simulink model "coif1_5_Level"  (R2021a)
settings: Solver=VariableStepAuto  StartTime=0.0  StopTime=8  RelTol=1e-3
undefined symbols (not defined in the file): lambda2
libraries: dspsigops x11, dspquant2 x1
(part 2 of 3)

== system coif1_5_Level/2nd_Level_Decomp/LoD_Even ==
  In_LoD_e : Inport  OutDataTypeStr=double  SampleTime=1/44100
  Add : Sum  AccumDataTypeStr=double  OutDataTypeStr=double  LockScale=on
  Add1 : Sum  AccumDataTypeStr=double  OutDataTypeStr=double  LockScale=on
  Delay{,1..3} (4 alike) : Delay  DelayLength=1  SampleTime=1/44100
  LoD_0 : Constant  Value=-0.015655728  OutDataTypeStr=double  SampleTime=1/44100
  LoD_2 : Constant  Value=0.384864847  OutDataTypeStr=double  SampleTime=1/44100
  LoD_4 : Constant  Value=0.337897662  OutDataTypeStr=double  SampleTime=1/44100
  Multiply : Product  OutDataTypeStr=double  LockScale=on
  Multiply1 : Product  OutDataTypeStr=double  LockScale=on
  Multiply2 : Product  OutDataTypeStr=double  LockScale=on
  Rate Transition : RateTransition  OutPortSampleTime=1/44100
  Rate Transition1 : RateTransition  OutPortSampleTime=1/44100
  Out_LoD_e : Outport  OutDataTypeStr=double  SampleTime=1/44100  VectorParamsAs1DForOutWhenUnconnected=off
  wires:
  In_LoD_e/1 -> Delay/1, Multiply/2
  Delay3/1 -> Add/2
  LoD_2/1 -> Multiply1/1
  Multiply/1 -> Add/1
  Rate Transition/1 -> Delay1/1, Multiply1/2
  LoD_4/1 -> Multiply2/1
  Delay2/1 -> Add1/2
  Multiply1/1 -> Add1/1
  Multiply2/1 -> Delay2/1
  Add1/1 -> Delay3/1
  Rate Transition1/1 -> Multiply2/2
  Add/1 -> Out_LoD_e/1
  Delay1/1 -> Rate Transition1/1
  LoD_0/1 -> Multiply/1
  Delay/1 -> Rate Transition/1

== system coif1_5_Level/2nd_Level_Decomp/LoD_Odd ==
  In_LoD_o : Inport  OutDataTypeStr=double  SampleTime=1/44100
  Add : Sum  AccumDataTypeStr=double  OutDataTypeStr=double  LockScale=on
  Add1 : Sum  AccumDataTypeStr=double  OutDataTypeStr=double  LockScale=on
  Delay{,1..3} (4 alike) : Delay  DelayLength=1  SampleTime=1/44100
  LoD_1 : Constant  Value=-0.07273262  OutDataTypeStr=double  SampleTime=1/44100
  LoD_3 : Constant  Value=0.85257202  OutDataTypeStr=double  SampleTime=1/44100
  LoD_5 : Constant  Value=-0.07273262  OutDataTypeStr=double  SampleTime=1/44100
  Multiply : Product  OutDataTypeStr=double  LockScale=on
  Multiply1 : Product  OutDataTypeStr=double  LockScale=on
  Multiply2 : Product  OutDataTypeStr=double  LockScale=on
  Rate Transition : RateTransition  OutPortSampleTime=1/44100
  Rate Transition1 : RateTransition  OutPortSampleTime=1/44100
  Out_LoD_o : Outport  OutDataTypeStr=double  SampleTime=1/44100  VectorParamsAs1DForOutWhenUnconnected=off
  wires:
  In_LoD_o/1 -> Delay/1, Multiply/2
  Delay3/1 -> Add/2
  LoD_3/1 -> Multiply1/1
  Delay/1 -> Rate Transition/1
  Multiply/1 -> Add/1
  Rate Transition/1 -> Delay1/1, Multiply1/2
  LoD_5/1 -> Multiply2/1
  Delay2/1 -> Add1/2
  Multiply1/1 -> Add1/1
  Multiply2/1 -> Delay2/1
  Add1/1 -> Delay3/1
  Rate Transition1/1 -> Multiply2/2
  Add/1 -> Out_LoD_o/1
  Delay1/1 -> Rate Transition1/1
  LoD_1/1 -> Multiply/1

== system coif1_5_Level/2nd_Level_Recon/HiR_Even1 ==
  In_HiR_e : Inport  OutDataTypeStr=double  SampleTime=1/44100
  Add : Sum  AccumDataTypeStr=double  OutDataTypeStr=double  LockScale=on
  Add1 : Sum  AccumDataTypeStr=double  OutDataTypeStr=double  LockScale=on
  Delay{,1..3} (4 alike) : Delay  DelayLength=1  SampleTime=1/44100
  HiR_0 : Constant  Value=-0.015655728  OutDataTypeStr=double  SampleTime=1/44100
  HiR_2 : Constant  Value=0.384864847  OutDataTypeStr=double  SampleTime=1/44100
  HiR_4 : Constant  Value=0.337897662  OutDataTypeStr=double  SampleTime=1/44100
  Multiply : Product  OutDataTypeStr=double  LockScale=on
  Multiply1 : Product  OutDataTypeStr=double  LockScale=on
  Multiply2 : Product  OutDataTypeStr=double  LockScale=on
  Rate Transition : RateTransition  OutPortSampleTime=1/44100
  Rate Transition1 : RateTransition  OutPortSampleTime=1/44100
  Out_HiR_e : Outport  OutDataTypeStr=double  SampleTime=1/44100  VectorParamsAs1DForOutWhenUnconnected=off
  wires:
  In_HiR_e/1 -> Multiply/2, Delay/1
  Delay/1 -> Rate Transition/1
  Delay3/1 -> Add/2
  Multiply/1 -> Add/1
  HiR_0/1 -> Multiply/1
  HiR_2/1 -> Multiply1/1
  Rate Transition/1 -> Delay1/1, Multiply1/2
  Add/1 -> Out_HiR_e/1
  Delay1/1 -> Rate Transition1/1
  Rate Transition1/1 -> Multiply2/2
  Multiply2/1 -> Delay2/1
  Delay2/1 -> Add1/2
  Multiply1/1 -> Add1/1
  Add1/1 -> Delay3/1
  HiR_4/1 -> Multiply2/1

== system coif1_5_Level/2nd_Level_Recon/HiR_Odd1 ==
  In_HiR_o : Inport  OutDataTypeStr=double  SampleTime=1/44100
  Add1 : Sum  AccumDataTypeStr=double  OutDataTypeStr=double  LockScale=on
  Add2 : Sum  AccumDataTypeStr=double  OutDataTypeStr=double  LockScale=on
  Delay{1..2,4..5} (4 alike) : Delay  DelayLength=1  SampleTime=1/44100
  HiR_1 : Constant  Value=0.07273262  OutDataTypeStr=double  SampleTime=1/44100
  HiR_3 : Constant  Value=-0.85257202  OutDataTypeStr=double  SampleTime=1/44100
  HiR_5 : Constant  Value=0.07273262  OutDataTypeStr=double  SampleTime=1/44100
  Multiply2 : Product  OutDataTypeStr=double  LockScale=on
  Multiply3 : Product  OutDataTypeStr=double  LockScale=on
  Multiply4 : Product  OutDataTypeStr=double  LockScale=on
  Rate Transition1 : RateTransition  OutPortSampleTime=1/44100
  Rate Transition2 : RateTransition  OutPortSampleTime=1/44100
  Out_HiR_o : Outport  OutDataTypeStr=double  SampleTime=1/44100  VectorParamsAs1DForOutWhenUnconnected=off
  wires:
  HiR_5/1 -> Multiply4/1
  Add1/1 -> Out_HiR_o/1
  Rate Transition2/1 -> Multiply4/2
  Rate Transition1/1 -> Delay2/1, Multiply3/2
  Multiply4/1 -> Delay4/1
  Add2/1 -> Delay5/1
  Multiply3/1 -> Add2/1
  Delay4/1 -> Add2/2
  Multiply2/1 -> Add1/1
  Delay2/1 -> Rate Transition2/1
  In_HiR_o/1 -> Multiply2/2, Delay1/1
  Delay1/1 -> Rate Transition1/1
  Delay5/1 -> Add1/2
  HiR_1/1 -> Multiply2/1
  HiR_3/1 -> Multiply3/1

== system coif1_5_Level/2nd_Level_Recon/LoR_Even1 ==
  In_LoR_e : Inport  OutDataTypeStr=double  SampleTime=1/44100
  Add1 : Sum  AccumDataTypeStr=double  OutDataTypeStr=double  LockScale=on
  Add2 : Sum  AccumDataTypeStr=double  OutDataTypeStr=double  LockScale=on
  Delay{1..2,4..5} (4 alike) : Delay  DelayLength=1  SampleTime=1/44100
  LoR_0 : Constant  Value=-0.07273262  OutDataTypeStr=double  SampleTime=1/44100
  LoR_2 : Constant  Value=0.85257202  OutDataTypeStr=double  SampleTime=1/44100
  LoR_4 : Constant  Value=-0.07273262  OutDataTypeStr=double  SampleTime=1/44100
  Multiply2 : Product  OutDataTypeStr=double  LockScale=on
  Multiply3 : Product  OutDataTypeStr=double  LockScale=on
  Multiply4 : Product  OutDataTypeStr=double  LockScale=on
  Rate Transition1 : RateTransition  OutPortSampleTime=1/44100
  Rate Transition2 : RateTransition  OutPortSampleTime=1/44100
  Out_LoR_e : Outport  OutDataTypeStr=double  SampleTime=1/44100  VectorParamsAs1DForOutWhenUnconnected=off
  wires:
  Add2/1 -> Delay5/1
  Delay2/1 -> Rate Transition2/1
  Add1/1 -> Out_LoR_e/1
  Multiply3/1 -> Add2/1
  Delay5/1 -> Add1/2
  Delay1/1 -> Rate Transition1/1
  Multiply2/1 -> Add1/1
  Delay4/1 -> Add2/2
  Multiply4/1 -> Delay4/1
  Rate Transition2/1 -> Multiply4/2
  In_LoR_e/1 -> Multiply2/2, Delay1/1
  Rate Transition1/1 -> Delay2/1, Multiply3/2
  LoR_4/1 -> Multiply4/1
  LoR_2/1 -> Multiply3/1
  LoR_0/1 -> Multiply2/1

== system coif1_5_Level/2nd_Level_Recon/LoR_Odd1 ==
  In_LoR_o : Inport  OutDataTypeStr=double  SampleTime=1/44100
  Add1 : Sum  AccumDataTypeStr=double  OutDataTypeStr=double  LockScale=on
  Add2 : Sum  AccumDataTypeStr=double  OutDataTypeStr=double  LockScale=on
  Delay{1..2,4..5} (4 alike) : Delay  DelayLength=1  SampleTime=1/44100
  LoR_1 : Constant  Value=0.337897662  OutDataTypeStr=double  SampleTime=1/44100
  LoR_3 : Constant  Value=0.384864847  OutDataTypeStr=double  SampleTime=1/44100
  LoR_5 : Constant  Value=-0.015655728  OutDataTypeStr=double  SampleTime=1/44100
  Multiply2 : Product  OutDataTypeStr=double  LockScale=on
  Multiply3 : Product  OutDataTypeStr=double  LockScale=on
  Multiply4 : Product  OutDataTypeStr=double  LockScale=on
  Rate Transition1 : RateTransition  OutPortSampleTime=1/44100
  Rate Transition2 : RateTransition  OutPortSampleTime=1/44100
  Out_HiR_o : Outport  OutDataTypeStr=double  SampleTime=1/44100  VectorParamsAs1DForOutWhenUnconnected=off
  wires:
  LoR_5/1 -> Multiply4/1
  In_LoR_o/1 -> Multiply2/2, Delay1/1
  LoR_3/1 -> Multiply3/1
  Delay2/1 -> Rate Transition2/1
  Add2/1 -> Delay5/1
  Multiply3/1 -> Add2/1
  Multiply2/1 -> Add1/1
  Delay4/1 -> Add2/2
  Rate Transition1/1 -> Delay2/1, Multiply3/2
  LoR_1/1 -> Multiply2/1
  Delay5/1 -> Add1/2
  Rate Transition2/1 -> Multiply4/2
  Delay1/1 -> Rate Transition1/1
  Multiply4/1 -> Delay4/1
  Add1/1 -> Out_HiR_o/1

== system coif1_5_Level/3rd_Level_Decomp/HiD_Even ==
  In_HiD_e : Inport  OutDataTypeStr=double  SampleTime=1/44100
  Add : Sum  AccumDataTypeStr=double  OutDataTypeStr=double  LockScale=on
  Add1 : Sum  AccumDataTypeStr=double  OutDataTypeStr=double  LockScale=on
  Delay{,1..3} (4 alike) : Delay  DelayLength=1  SampleTime=1/44100
  HiD_0 : Constant  Value=0.07273262  OutDataTypeStr=double  SampleTime=1/44100
  HiD_2 : Constant  Value=-0.85257202  OutDataTypeStr=double  SampleTime=1/44100
  HiD_4 : Constant  Value=0.07273262  OutDataTypeStr=double  SampleTime=1/44100
  Multiply : Product  OutDataTypeStr=double  LockScale=on
  Multiply1 : Product  OutDataTypeStr=double  LockScale=on
  Multiply2 : Product  OutDataTypeStr=double  LockScale=on
  Rate Transition : RateTransition  OutPortSampleTime=1/44100
  Rate Transition1 : RateTransition  OutPortSampleTime=1/44100
  Out_HiD_e : Outport  OutDataTypeStr=double  SampleTime=1/44100  VectorParamsAs1DForOutWhenUnconnected=off
  wires:
  In_HiD_e/1 -> Delay/1, Multiply/2
  Delay3/1 -> Add/2
  HiD_2/1 -> Multiply1/1
  Delay/1 -> Rate Transition/1
  Multiply/1 -> Add/1
  Rate Transition/1 -> Delay1/1, Multiply1/2
  HiD_4/1 -> Multiply2/1
  Delay2/1 -> Add1/2
  Multiply1/1 -> Add1/1
  Multiply2/1 -> Delay2/1
  Add1/1 -> Delay3/1
  Rate Transition1/1 -> Multiply2/2
  Add/1 -> Out_HiD_e/1
  Delay1/1 -> Rate Transition1/1
  HiD_0/1 -> Multiply/1

== system coif1_5_Level/3rd_Level_Decomp/HiD_Odd ==
  In_HiD_o : Inport  OutDataTypeStr=double  SampleTime=1/44100
  Add : Sum  AccumDataTypeStr=double  OutDataTypeStr=double
  Add1 : Sum  AccumDataTypeStr=double  OutDataTypeStr=double  LockScale=on
  Delay{,1..3} (4 alike) : Delay  DelayLength=1  SampleTime=1/44100
  HiD_1 : Constant  Value=0.337897662  OutDataTypeStr=double  SampleTime=1/44100
  HiD_3 : Constant  Value=0.384864847  OutDataTypeStr=fixdt(1,16,12)  SampleTime=1/44100
  HiD_5 : Constant  Value=-0.015655728  OutDataTypeStr=fixdt(1,16,12)  SampleTime=1/44100
  Multiply : Product  OutDataTypeStr=double  LockScale=on
  Multiply1 : Product  OutDataTypeStr=double  LockScale=on
  Multiply2 : Product  OutDataTypeStr=double  LockScale=on
  Rate Transition : RateTransition  OutPortSampleTime=1/44100
  Rate Transition1 : RateTransition  OutPortSampleTime=1/44100
  Out_HiD_o : Outport  OutDataTypeStr=double  SampleTime=1/44100  VectorParamsAs1DForOutWhenUnconnected=off
  wires:
  In_HiD_o/1 -> Delay/1, Multiply/2
  Delay3/1 -> Add/2
  HiD_3/1 -> Multiply1/1
  Multiply/1 -> Add/1
  Rate Transition/1 -> Delay1/1, Multiply1/2
  Delay2/1 -> Add1/2
  Multiply1/1 -> Add1/1
  Multiply2/1 -> Delay2/1
  Add1/1 -> Delay3/1
  Rate Transition1/1 -> Multiply2/2
  Add/1 -> Out_HiD_o/1
  Delay1/1 -> Rate Transition1/1
  HiD_1/1 -> Multiply/1
  Delay/1 -> Rate Transition/1
  HiD_5/1 -> Multiply2/1

== system coif1_5_Level/3rd_Level_Decomp/LoD_Even ==
  In_LoD_e : Inport  OutDataTypeStr=double  SampleTime=1/44100
  Add : Sum  AccumDataTypeStr=double  OutDataTypeStr=double  LockScale=on
  Add1 : Sum  AccumDataTypeStr=double  OutDataTypeStr=double  LockScale=on
  Delay{,1..3} (4 alike) : Delay  DelayLength=1  SampleTime=1/44100
  LoD_0 : Constant  Value=-0.015655728  OutDataTypeStr=double  SampleTime=1/44100
  LoD_2 : Constant  Value=0.384864847  OutDataTypeStr=double  SampleTime=1/44100
  LoD_4 : Constant  Value=0.337897662  OutDataTypeStr=double  SampleTime=1/44100
  Multiply : Product  OutDataTypeStr=double  LockScale=on
  Multiply1 : Product  OutDataTypeStr=double  LockScale=on
  Multiply2 : Product  OutDataTypeStr=double  LockScale=on
  Rate Transition : RateTransition  OutPortSampleTime=1/44100
  Rate Transition1 : RateTransition  OutPortSampleTime=1/44100
  Out_LoD_e : Outport  OutDataTypeStr=double  SampleTime=1/44100  VectorParamsAs1DForOutWhenUnconnected=off
  wires:
  In_LoD_e/1 -> Delay/1, Multiply/2
  Delay3/1 -> Add/2
  LoD_2/1 -> Multiply1/1
  Multiply/1 -> Add/1
  Rate Transition/1 -> Delay1/1, Multiply1/2
  LoD_4/1 -> Multiply2/1
  Delay2/1 -> Add1/2
  Multiply1/1 -> Add1/1
  Multiply2/1 -> Delay2/1
  Add1/1 -> Delay3/1
  Rate Transition1/1 -> Multiply2/2
  Add/1 -> Out_LoD_e/1
  Delay1/1 -> Rate Transition1/1
  LoD_0/1 -> Multiply/1
  Delay/1 -> Rate Transition/1

== system coif1_5_Level/3rd_Level_Decomp/LoD_Odd ==
  In_LoD_o : Inport  OutDataTypeStr=double  SampleTime=1/44100
  Add : Sum  AccumDataTypeStr=double  OutDataTypeStr=double  LockScale=on
  Add1 : Sum  AccumDataTypeStr=double  OutDataTypeStr=double  LockScale=on
  Delay{,1..3} (4 alike) : Delay  DelayLength=1  SampleTime=1/44100
  LoD_1 : Constant  Value=-0.07273262  OutDataTypeStr=double  SampleTime=1/44100
  LoD_3 : Constant  Value=0.85257202  OutDataTypeStr=double  SampleTime=1/44100
  LoD_5 : Constant  Value=-0.07273262  OutDataTypeStr=double  SampleTime=1/44100
  Multiply : Product  OutDataTypeStr=double  LockScale=on
  Multiply1 : Product  OutDataTypeStr=double  LockScale=on
  Multiply2 : Product  OutDataTypeStr=double  LockScale=on
  Rate Transition : RateTransition  OutPortSampleTime=1/44100
  Rate Transition1 : RateTransition  OutPortSampleTime=1/44100
  Out_LoD_o : Outport  OutDataTypeStr=double  SampleTime=1/44100  VectorParamsAs1DForOutWhenUnconnected=off
  wires:
  In_LoD_o/1 -> Delay/1, Multiply/2
  Delay3/1 -> Add/2
  LoD_3/1 -> Multiply1/1
  Delay/1 -> Rate Transition/1
  Multiply/1 -> Add/1
  Rate Transition/1 -> Delay1/1, Multiply1/2
  LoD_5/1 -> Multiply2/1
  Delay2/1 -> Add1/2
  Multiply1/1 -> Add1/1
  Multiply2/1 -> Delay2/1
  Add1/1 -> Delay3/1
  Rate Transition1/1 -> Multiply2/2
  Add/1 -> Out_LoD_o/1
  Delay1/1 -> Rate Transition1/1
  LoD_1/1 -> Multiply/1

== system coif1_5_Level/3rd_Level_Recon/HiR_Even1 ==
  In_HiR_e : Inport  OutDataTypeStr=double  SampleTime=1/44100
  Add : Sum  AccumDataTypeStr=double  OutDataTypeStr=double  LockScale=on
  Add1 : Sum  AccumDataTypeStr=double  OutDataTypeStr=double  LockScale=on
  Delay{,1..3} (4 alike) : Delay  DelayLength=1  SampleTime=1/44100
  HiR_0 : Constant  Value=-0.015655728  OutDataTypeStr=double  SampleTime=1/44100
  HiR_2 : Constant  Value=0.384864847  OutDataTypeStr=double  SampleTime=1/44100
  HiR_4 : Constant  Value=0.337897662  OutDataTypeStr=double  SampleTime=1/44100
  Multiply : Product  OutDataTypeStr=double  LockScale=on
  Multiply1 : Product  OutDataTypeStr=double  LockScale=on
  Multiply2 : Product  OutDataTypeStr=double  LockScale=on
  Rate Transition : RateTransition  OutPortSampleTime=1/44100
  Rate Transition1 : RateTransition  OutPortSampleTime=1/44100
  Out_HiR_e : Outport  OutDataTypeStr=double  SampleTime=1/44100  VectorParamsAs1DForOutWhenUnconnected=off
  wires:
  In_HiR_e/1 -> Multiply/2, Delay/1
  Delay/1 -> Rate Transition/1
  Delay3/1 -> Add/2
  Multiply/1 -> Add/1
  HiR_0/1 -> Multiply/1
  HiR_2/1 -> Multiply1/1
  Rate Transition/1 -> Delay1/1, Multiply1/2
  Add/1 -> Out_HiR_e/1
  Delay1/1 -> Rate Transition1/1
  Rate Transition1/1 -> Multiply2/2
  Multiply2/1 -> Delay2/1
  Delay2/1 -> Add1/2
  Multiply1/1 -> Add1/1
  Add1/1 -> Delay3/1
  HiR_4/1 -> Multiply2/1

== system coif1_5_Level/3rd_Level_Recon/HiR_Odd1 ==
  In_HiR_o : Inport  OutDataTypeStr=double  SampleTime=1/44100
  Add1 : Sum  AccumDataTypeStr=double  OutDataTypeStr=double  LockScale=on
  Add2 : Sum  AccumDataTypeStr=double  OutDataTypeStr=double  LockScale=on
  Delay{1..2,4..5} (4 alike) : Delay  DelayLength=1  SampleTime=1/44100
  HiR_1 : Constant  Value=0.07273262  OutDataTypeStr=double  SampleTime=1/44100
  HiR_3 : Constant  Value=-0.85257202  OutDataTypeStr=double  SampleTime=1/44100
  HiR_5 : Constant  Value=0.07273262  OutDataTypeStr=double  SampleTime=1/44100
  Multiply2 : Product  OutDataTypeStr=double  LockScale=on
  Multiply3 : Product  OutDataTypeStr=double  LockScale=on
  Multiply4 : Product  OutDataTypeStr=double  LockScale=on
  Rate Transition1 : RateTransition  OutPortSampleTime=1/44100
  Rate Transition2 : RateTransition  OutPortSampleTime=1/44100
  Out_HiR_o : Outport  OutDataTypeStr=double  SampleTime=1/44100  VectorParamsAs1DForOutWhenUnconnected=off
  wires:
  HiR_5/1 -> Multiply4/1
  Add1/1 -> Out_HiR_o/1
  Rate Transition2/1 -> Multiply4/2
  Rate Transition1/1 -> Delay2/1, Multiply3/2
  Multiply4/1 -> Delay4/1
  Add2/1 -> Delay5/1
  Multiply3/1 -> Add2/1
  Delay4/1 -> Add2/2
  Multiply2/1 -> Add1/1
  Delay2/1 -> Rate Transition2/1
  In_HiR_o/1 -> Multiply2/2, Delay1/1
  Delay1/1 -> Rate Transition1/1
  Delay5/1 -> Add1/2
  HiR_1/1 -> Multiply2/1
  HiR_3/1 -> Multiply3/1

== system coif1_5_Level/3rd_Level_Recon/LoR_Even1 ==
  In_LoR_e : Inport  OutDataTypeStr=double  SampleTime=1/44100
  Add1 : Sum  AccumDataTypeStr=double  OutDataTypeStr=double  LockScale=on
  Add2 : Sum  AccumDataTypeStr=double  OutDataTypeStr=double  LockScale=on
  Delay{1..2,4..5} (4 alike) : Delay  DelayLength=1  SampleTime=1/44100
  LoR_0 : Constant  Value=-0.07273262  OutDataTypeStr=double  SampleTime=1/44100
  LoR_2 : Constant  Value=0.85257202  OutDataTypeStr=double  SampleTime=1/44100
  LoR_4 : Constant  Value=-0.07273262  OutDataTypeStr=double  SampleTime=1/44100
  Multiply2 : Product  OutDataTypeStr=double  LockScale=on
  Multiply3 : Product  OutDataTypeStr=double  LockScale=on
  Multiply4 : Product  OutDataTypeStr=double  LockScale=on
  Rate Transition1 : RateTransition  OutPortSampleTime=1/44100
  Rate Transition2 : RateTransition  OutPortSampleTime=1/44100
  Out_LoR_e : Outport  OutDataTypeStr=double  SampleTime=1/44100  VectorParamsAs1DForOutWhenUnconnected=off
  wires:
  Add2/1 -> Delay5/1
  Delay2/1 -> Rate Transition2/1
  Add1/1 -> Out_LoR_e/1
  Multiply3/1 -> Add2/1
  Delay5/1 -> Add1/2
  Delay1/1 -> Rate Transition1/1
  Multiply2/1 -> Add1/1
  Delay4/1 -> Add2/2
  Multiply4/1 -> Delay4/1
  Rate Transition2/1 -> Multiply4/2
  In_LoR_e/1 -> Multiply2/2, Delay1/1
  Rate Transition1/1 -> Delay2/1, Multiply3/2
  LoR_4/1 -> Multiply4/1
  LoR_2/1 -> Multiply3/1
  LoR_0/1 -> Multiply2/1

== system coif1_5_Level/3rd_Level_Recon/LoR_Odd1 ==
  In_LoR_o : Inport  OutDataTypeStr=double  SampleTime=1/44100
  Add1 : Sum  AccumDataTypeStr=double  OutDataTypeStr=double  LockScale=on
  Add2 : Sum  AccumDataTypeStr=double  OutDataTypeStr=double  LockScale=on
  Delay{1..2,4..5} (4 alike) : Delay  DelayLength=1  SampleTime=1/44100
  LoR_1 : Constant  Value=0.337897662  OutDataTypeStr=double  SampleTime=1/44100
  LoR_3 : Constant  Value=0.384864847  OutDataTypeStr=double  SampleTime=1/44100
  LoR_5 : Constant  Value=-0.015655728  OutDataTypeStr=double  SampleTime=1/44100
  Multiply2 : Product  OutDataTypeStr=double  LockScale=on
  Multiply3 : Product  OutDataTypeStr=double  LockScale=on
  Multiply4 : Product  OutDataTypeStr=double  LockScale=on
  Rate Transition1 : RateTransition  OutPortSampleTime=1/44100
  Rate Transition2 : RateTransition  OutPortSampleTime=1/44100
  Out_HiR_o : Outport  OutDataTypeStr=double  SampleTime=1/44100  VectorParamsAs1DForOutWhenUnconnected=off
  wires:
  LoR_5/1 -> Multiply4/1
  In_LoR_o/1 -> Multiply2/2, Delay1/1
  LoR_3/1 -> Multiply3/1
  Delay2/1 -> Rate Transition2/1
  Add2/1 -> Delay5/1
  Multiply3/1 -> Add2/1
  Multiply2/1 -> Add1/1
  Delay4/1 -> Add2/2
  Rate Transition1/1 -> Delay2/1, Multiply3/2
  LoR_1/1 -> Multiply2/1
  Delay5/1 -> Add1/2
  Rate Transition2/1 -> Multiply4/2
  Delay1/1 -> Rate Transition1/1
  Multiply4/1 -> Delay4/1
  Add1/1 -> Out_HiR_o/1

== system coif1_5_Level/4th_Level_Decomp/HiD_Even ==
  In_HiD_e : Inport  OutDataTypeStr=double  SampleTime=1/44100
  Add : Sum  AccumDataTypeStr=double  OutDataTypeStr=double  LockScale=on
  Add1 : Sum  AccumDataTypeStr=double  OutDataTypeStr=double  LockScale=on
  Delay{,1..3} (4 alike) : Delay  DelayLength=1  SampleTime=1/44100
  HiD_0 : Constant  Value=0.07273262  OutDataTypeStr=double  SampleTime=1/44100
  HiD_2 : Constant  Value=-0.85257202  OutDataTypeStr=double  SampleTime=1/44100
  HiD_4 : Constant  Value=0.07273262  OutDataTypeStr=double  SampleTime=1/44100
  Multiply : Product  OutDataTypeStr=double  LockScale=on
  Multiply1 : Product  OutDataTypeStr=double  LockScale=on
  Multiply2 : Product  OutDataTypeStr=double  LockScale=on
  Rate Transition : RateTransition  OutPortSampleTime=1/44100
  Rate Transition1 : RateTransition  OutPortSampleTime=1/44100
  Out_HiD_e : Outport  OutDataTypeStr=double  SampleTime=1/44100  VectorParamsAs1DForOutWhenUnconnected=off
  wires:
  In_HiD_e/1 -> Delay/1, Multiply/2
  Delay3/1 -> Add/2
  HiD_2/1 -> Multiply1/1
  Delay/1 -> Rate Transition/1
  Multiply/1 -> Add/1
  Rate Transition/1 -> Delay1/1, Multiply1/2
  HiD_4/1 -> Multiply2/1
  Delay2/1 -> Add1/2
  Multiply1/1 -> Add1/1
  Multiply2/1 -> Delay2/1
  Add1/1 -> Delay3/1
  Rate Transition1/1 -> Multiply2/2
  Add/1 -> Out_HiD_e/1
  Delay1/1 -> Rate Transition1/1
  HiD_0/1 -> Multiply/1

== system coif1_5_Level/4th_Level_Decomp/HiD_Odd ==
  In_HiD_o : Inport  OutDataTypeStr=double  SampleTime=1/44100
  Add : Sum  AccumDataTypeStr=double  OutDataTypeStr=double
  Add1 : Sum  AccumDataTypeStr=double  OutDataTypeStr=double  LockScale=on
  Delay{,1..3} (4 alike) : Delay  DelayLength=1  SampleTime=1/44100
  HiD_1 : Constant  Value=0.337897662  OutDataTypeStr=double  SampleTime=1/44100
  HiD_3 : Constant  Value=0.384864847  OutDataTypeStr=fixdt(1,16,12)  SampleTime=1/44100
  HiD_5 : Constant  Value=-0.015655728  OutDataTypeStr=fixdt(1,16,12)  SampleTime=1/44100
  Multiply : Product  OutDataTypeStr=double  LockScale=on
  Multiply1 : Product  OutDataTypeStr=double  LockScale=on
  Multiply2 : Product  OutDataTypeStr=double  LockScale=on
  Rate Transition : RateTransition  OutPortSampleTime=1/44100
  Rate Transition1 : RateTransition  OutPortSampleTime=1/44100
  Out_HiD_o : Outport  OutDataTypeStr=double  SampleTime=1/44100  VectorParamsAs1DForOutWhenUnconnected=off
  wires:
  In_HiD_o/1 -> Delay/1, Multiply/2
  Delay3/1 -> Add/2
  HiD_3/1 -> Multiply1/1
  Multiply/1 -> Add/1
  Rate Transition/1 -> Delay1/1, Multiply1/2
  Delay2/1 -> Add1/2
  Multiply1/1 -> Add1/1
  Multiply2/1 -> Delay2/1
  Add1/1 -> Delay3/1
  Rate Transition1/1 -> Multiply2/2
  Add/1 -> Out_HiD_o/1
  Delay1/1 -> Rate Transition1/1
  HiD_1/1 -> Multiply/1
  Delay/1 -> Rate Transition/1
  HiD_5/1 -> Multiply2/1

== system coif1_5_Level/4th_Level_Decomp/LoD_Even ==
  In_LoD_e : Inport  OutDataTypeStr=double  SampleTime=1/44100
  Add : Sum  AccumDataTypeStr=double  OutDataTypeStr=double  LockScale=on
  Add1 : Sum  AccumDataTypeStr=double  OutDataTypeStr=double  LockScale=on
  Delay{,1..3} (4 alike) : Delay  DelayLength=1  SampleTime=1/44100
  LoD_0 : Constant  Value=-0.015655728  OutDataTypeStr=double  SampleTime=1/44100
  LoD_2 : Constant  Value=0.384864847  OutDataTypeStr=double  SampleTime=1/44100
  LoD_4 : Constant  Value=0.337897662  OutDataTypeStr=double  SampleTime=1/44100
  Multiply : Product  OutDataTypeStr=double  LockScale=on
  Multiply1 : Product  OutDataTypeStr=double  LockScale=on
  Multiply2 : Product  OutDataTypeStr=double  LockScale=on
  Rate Transition : RateTransition  OutPortSampleTime=1/44100
  Rate Transition1 : RateTransition  OutPortSampleTime=1/44100
  Out_LoD_e : Outport  OutDataTypeStr=double  SampleTime=1/44100  VectorParamsAs1DForOutWhenUnconnected=off
  wires:
  In_LoD_e/1 -> Delay/1, Multiply/2
  Delay3/1 -> Add/2
  LoD_2/1 -> Multiply1/1
  Multiply/1 -> Add/1
  Rate Transition/1 -> Delay1/1, Multiply1/2
  LoD_4/1 -> Multiply2/1
  Delay2/1 -> Add1/2
  Multiply1/1 -> Add1/1
  Multiply2/1 -> Delay2/1
  Add1/1 -> Delay3/1
  Rate Transition1/1 -> Multiply2/2
  Add/1 -> Out_LoD_e/1
  Delay1/1 -> Rate Transition1/1
  LoD_0/1 -> Multiply/1
  Delay/1 -> Rate Transition/1

== system coif1_5_Level/4th_Level_Decomp/LoD_Odd ==
  In_LoD_o : Inport  OutDataTypeStr=double  SampleTime=1/44100
  Add : Sum  AccumDataTypeStr=double  OutDataTypeStr=double  LockScale=on
  Add1 : Sum  AccumDataTypeStr=double  OutDataTypeStr=double  LockScale=on
  Delay{,1..3} (4 alike) : Delay  DelayLength=1  SampleTime=1/44100
  LoD_1 : Constant  Value=-0.07273262  OutDataTypeStr=double  SampleTime=1/44100
  LoD_3 : Constant  Value=0.85257202  OutDataTypeStr=double  SampleTime=1/44100
  LoD_5 : Constant  Value=-0.07273262  OutDataTypeStr=double  SampleTime=1/44100
  Multiply : Product  OutDataTypeStr=double  LockScale=on
  Multiply1 : Product  OutDataTypeStr=double  LockScale=on
  Multiply2 : Product  OutDataTypeStr=double  LockScale=on
  Rate Transition : RateTransition  OutPortSampleTime=1/44100
  Rate Transition1 : RateTransition  OutPortSampleTime=1/44100
  Out_LoD_o : Outport  OutDataTypeStr=double  SampleTime=1/44100  VectorParamsAs1DForOutWhenUnconnected=off
  wires:
  In_LoD_o/1 -> Delay/1, Multiply/2
  Delay3/1 -> Add/2
  LoD_3/1 -> Multiply1/1
  Delay/1 -> Rate Transition/1
  Multiply/1 -> Add/1
  Rate Transition/1 -> Delay1/1, Multiply1/2
  LoD_5/1 -> Multiply2/1
  Delay2/1 -> Add1/2
  Multiply1/1 -> Add1/1
  Multiply2/1 -> Delay2/1
  Add1/1 -> Delay3/1
  Rate Transition1/1 -> Multiply2/2
  Add/1 -> Out_LoD_o/1
  Delay1/1 -> Rate Transition1/1
  LoD_1/1 -> Multiply/1

== system coif1_5_Level/4th_Level_Recon/HiR_Even1 ==
  In_HiR_e : Inport  OutDataTypeStr=double  SampleTime=1/44100
  Add : Sum  AccumDataTypeStr=double  OutDataTypeStr=double  LockScale=on
  Add1 : Sum  AccumDataTypeStr=double  OutDataTypeStr=double  LockScale=on
  Delay{,1..3} (4 alike) : Delay  DelayLength=1  SampleTime=1/44100
  HiR_0 : Constant  Value=-0.015655728  OutDataTypeStr=double  SampleTime=1/44100
  HiR_2 : Constant  Value=0.384864847  OutDataTypeStr=double  SampleTime=1/44100
  HiR_4 : Constant  Value=0.337897662  OutDataTypeStr=double  SampleTime=1/44100
  Multiply : Product  OutDataTypeStr=double  LockScale=on
  Multiply1 : Product  OutDataTypeStr=double  LockScale=on
  Multiply2 : Product  OutDataTypeStr=double  LockScale=on
  Rate Transition : RateTransition  OutPortSampleTime=1/44100
  Rate Transition1 : RateTransition  OutPortSampleTime=1/44100
  Out_HiR_e : Outport  OutDataTypeStr=double  SampleTime=1/44100  VectorParamsAs1DForOutWhenUnconnected=off
  wires:
  In_HiR_e/1 -> Multiply/2, Delay/1
  Delay/1 -> Rate Transition/1
  Delay3/1 -> Add/2
  Multiply/1 -> Add/1
  HiR_0/1 -> Multiply/1
  HiR_2/1 -> Multiply1/1
  Rate Transition/1 -> Delay1/1, Multiply1/2
  Add/1 -> Out_HiR_e/1
  Delay1/1 -> Rate Transition1/1
  Rate Transition1/1 -> Multiply2/2
  Multiply2/1 -> Delay2/1
  Delay2/1 -> Add1/2
  Multiply1/1 -> Add1/1
  Add1/1 -> Delay3/1
  HiR_4/1 -> Multiply2/1

== system coif1_5_Level/4th_Level_Recon/HiR_Odd1 ==
  In_HiR_o : Inport  OutDataTypeStr=double  SampleTime=1/44100
  Add1 : Sum  AccumDataTypeStr=double  OutDataTypeStr=double  LockScale=on
  Add2 : Sum  AccumDataTypeStr=double  OutDataTypeStr=double  LockScale=on
  Delay{1..2,4..5} (4 alike) : Delay  DelayLength=1  SampleTime=1/44100
  HiR_1 : Constant  Value=0.07273262  OutDataTypeStr=double  SampleTime=1/44100
  HiR_3 : Constant  Value=-0.85257202  OutDataTypeStr=double  SampleTime=1/44100
  HiR_5 : Constant  Value=0.07273262  OutDataTypeStr=double  SampleTime=1/44100
  Multiply2 : Product  OutDataTypeStr=double  LockScale=on
  Multiply3 : Product  OutDataTypeStr=double  LockScale=on
  Multiply4 : Product  OutDataTypeStr=double  LockScale=on
  Rate Transition1 : RateTransition  OutPortSampleTime=1/44100
  Rate Transition2 : RateTransition  OutPortSampleTime=1/44100
  Out_HiR_o : Outport  OutDataTypeStr=double  SampleTime=1/44100  VectorParamsAs1DForOutWhenUnconnected=off
  wires:
  HiR_5/1 -> Multiply4/1
  Add1/1 -> Out_HiR_o/1
  Rate Transition2/1 -> Multiply4/2
  Rate Transition1/1 -> Delay2/1, Multiply3/2
  Multiply4/1 -> Delay4/1
  Add2/1 -> Delay5/1
  Multiply3/1 -> Add2/1
  Delay4/1 -> Add2/2
  Multiply2/1 -> Add1/1
  Delay2/1 -> Rate Transition2/1
  In_HiR_o/1 -> Multiply2/2, Delay1/1
  Delay1/1 -> Rate Transition1/1
  Delay5/1 -> Add1/2
  HiR_1/1 -> Multiply2/1
  HiR_3/1 -> Multiply3/1

== system coif1_5_Level/4th_Level_Recon/LoR_Even1 ==
  In_LoR_e : Inport  OutDataTypeStr=double  SampleTime=1/44100
  Add1 : Sum  AccumDataTypeStr=double  OutDataTypeStr=double  LockScale=on
  Add2 : Sum  AccumDataTypeStr=double  OutDataTypeStr=double  LockScale=on
  Delay{1..2,4..5} (4 alike) : Delay  DelayLength=1  SampleTime=1/44100
  LoR_0 : Constant  Value=-0.07273262  OutDataTypeStr=double  SampleTime=1/44100
  LoR_2 : Constant  Value=0.85257202  OutDataTypeStr=double  SampleTime=1/44100
  LoR_4 : Constant  Value=-0.07273262  OutDataTypeStr=double  SampleTime=1/44100
  Multiply2 : Product  OutDataTypeStr=double  LockScale=on
  Multiply3 : Product  OutDataTypeStr=double  LockScale=on
  Multiply4 : Product  OutDataTypeStr=double  LockScale=on
  Rate Transition1 : RateTransition  OutPortSampleTime=1/44100
  Rate Transition2 : RateTransition  OutPortSampleTime=1/44100
  Out_LoR_e : Outport  OutDataTypeStr=double  SampleTime=1/44100  VectorParamsAs1DForOutWhenUnconnected=off
  wires:
  Add2/1 -> Delay5/1
  Delay2/1 -> Rate Transition2/1
  Add1/1 -> Out_LoR_e/1
  Multiply3/1 -> Add2/1
  Delay5/1 -> Add1/2
  Delay1/1 -> Rate Transition1/1
  Multiply2/1 -> Add1/1
  Delay4/1 -> Add2/2
  Multiply4/1 -> Delay4/1
  Rate Transition2/1 -> Multiply4/2
  In_LoR_e/1 -> Multiply2/2, Delay1/1
  Rate Transition1/1 -> Delay2/1, Multiply3/2
  LoR_4/1 -> Multiply4/1
  LoR_2/1 -> Multiply3/1
  LoR_0/1 -> Multiply2/1

== system coif1_5_Level/4th_Level_Recon/LoR_Odd1 ==
  In_LoR_o : Inport  OutDataTypeStr=double  SampleTime=1/44100
  Add1 : Sum  AccumDataTypeStr=double  OutDataTypeStr=double  LockScale=on
  Add2 : Sum  AccumDataTypeStr=double  OutDataTypeStr=double  LockScale=on
  Delay{1..2,4..5} (4 alike) : Delay  DelayLength=1  SampleTime=1/44100
  LoR_1 : Constant  Value=0.337897662  OutDataTypeStr=double  SampleTime=1/44100
  LoR_3 : Constant  Value=0.384864847  OutDataTypeStr=double  SampleTime=1/44100
  LoR_5 : Constant  Value=-0.015655728  OutDataTypeStr=double  SampleTime=1/44100
  Multiply2 : Product  OutDataTypeStr=double  LockScale=on
  Multiply3 : Product  OutDataTypeStr=double  LockScale=on
  Multiply4 : Product  OutDataTypeStr=double  LockScale=on
  Rate Transition1 : RateTransition  OutPortSampleTime=1/44100
  Rate Transition2 : RateTransition  OutPortSampleTime=1/44100
  Out_HiR_o : Outport  OutDataTypeStr=double  SampleTime=1/44100  VectorParamsAs1DForOutWhenUnconnected=off
  wires:
  LoR_5/1 -> Multiply4/1
  In_LoR_o/1 -> Multiply2/2, Delay1/1
  LoR_3/1 -> Multiply3/1
  Delay2/1 -> Rate Transition2/1
  Add2/1 -> Delay5/1
  Multiply3/1 -> Add2/1
  Multiply2/1 -> Add1/1
  Delay4/1 -> Add2/2
  Rate Transition1/1 -> Delay2/1, Multiply3/2
  LoR_1/1 -> Multiply2/1
  Delay5/1 -> Add1/2
  Rate Transition2/1 -> Multiply4/2
  Delay1/1 -> Rate Transition1/1
  Multiply4/1 -> Delay4/1
  Add1/1 -> Out_HiR_o/1

== system coif1_5_Level/5th_Level_Decomp/HiD_Even ==
  In_HiD_e : Inport  OutDataTypeStr=double  SampleTime=1/44100
  Add : Sum  AccumDataTypeStr=double  OutDataTypeStr=double  LockScale=on
  Add1 : Sum  AccumDataTypeStr=double  OutDataTypeStr=double  LockScale=on
  Delay{,1..3} (4 alike) : Delay  DelayLength=1  SampleTime=1/44100
  HiD_0 : Constant  Value=0.07273262  OutDataTypeStr=double  SampleTime=1/44100
  HiD_2 : Constant  Value=-0.85257202  OutDataTypeStr=double  SampleTime=1/44100
  HiD_4 : Constant  Value=0.07273262  OutDataTypeStr=double  SampleTime=1/44100
  Multiply : Product  OutDataTypeStr=double  LockScale=on
  Multiply1 : Product  OutDataTypeStr=double  LockScale=on
  Multiply2 : Product  OutDataTypeStr=double  LockScale=on
  Rate Transition : RateTransition  OutPortSampleTime=1/44100
  Rate Transition1 : RateTransition  OutPortSampleTime=1/44100
  Out_HiD_e : Outport  OutDataTypeStr=double  SampleTime=1/44100  VectorParamsAs1DForOutWhenUnconnected=off
  wires:
  In_HiD_e/1 -> Delay/1, Multiply/2
  Delay3/1 -> Add/2
  HiD_2/1 -> Multiply1/1
  Delay/1 -> Rate Transition/1
  Multiply/1 -> Add/1
  Rate Transition/1 -> Delay1/1, Multiply1/2
  HiD_4/1 -> Multiply2/1
  Delay2/1 -> Add1/2
  Multiply1/1 -> Add1/1
  Multiply2/1 -> Delay2/1
  Add1/1 -> Delay3/1
  Rate Transition1/1 -> Multiply2/2
  Add/1 -> Out_HiD_e/1
  Delay1/1 -> Rate Transition1/1
  HiD_0/1 -> Multiply/1

== system coif1_5_Level/5th_Level_Decomp/HiD_Odd ==
  In_HiD_o : Inport  OutDataTypeStr=double  SampleTime=1/44100
  Add : Sum  AccumDataTypeStr=double  OutDataTypeStr=double
  Add1 : Sum  AccumDataTypeStr=double  OutDataTypeStr=double  LockScale=on
  Delay{,1..3} (4 alike) : Delay  DelayLength=1  SampleTime=1/44100
  HiD_1 : Constant  Value=0.337897662  OutDataTypeStr=double  SampleTime=1/44100
  HiD_3 : Constant  Value=0.384864847  OutDataTypeStr=fixdt(1,16,12)  SampleTime=1/44100
  HiD_5 : Constant  Value=-0.015655728  OutDataTypeStr=fixdt(1,16,12)  SampleTime=1/44100
  Multiply : Product  OutDataTypeStr=double  LockScale=on
  Multiply1 : Product  OutDataTypeStr=double  LockScale=on
  Multiply2 : Product  OutDataTypeStr=double  LockScale=on
  Rate Transition : RateTransition  OutPortSampleTime=1/44100
  Rate Transition1 : RateTransition  OutPortSampleTime=1/44100
  Out_HiD_o : Outport  OutDataTypeStr=double  SampleTime=1/44100  VectorParamsAs1DForOutWhenUnconnected=off
  wires:
  In_HiD_o/1 -> Delay/1, Multiply/2
  Delay3/1 -> Add/2
  HiD_3/1 -> Multiply1/1
  Multiply/1 -> Add/1
  Rate Transition/1 -> Delay1/1, Multiply1/2
  Delay2/1 -> Add1/2
  Multiply1/1 -> Add1/1
  Multiply2/1 -> Delay2/1
  Add1/1 -> Delay3/1
  Rate Transition1/1 -> Multiply2/2
  Add/1 -> Out_HiD_o/1
  Delay1/1 -> Rate Transition1/1
  HiD_1/1 -> Multiply/1
  Delay/1 -> Rate Transition/1
  HiD_5/1 -> Multiply2/1

== system coif1_5_Level/5th_Level_Decomp/LoD_Even ==
  In_LoD_e : Inport  OutDataTypeStr=double  SampleTime=1/44100
  Add : Sum  AccumDataTypeStr=double  OutDataTypeStr=double  LockScale=on
  Add1 : Sum  AccumDataTypeStr=double  OutDataTypeStr=double  LockScale=on
  Delay{,1..3} (4 alike) : Delay  DelayLength=1  SampleTime=1/44100
  LoD_0 : Constant  Value=-0.015655728  OutDataTypeStr=double  SampleTime=1/44100
  LoD_2 : Constant  Value=0.384864847  OutDataTypeStr=double  SampleTime=1/44100
  LoD_4 : Constant  Value=0.337897662  OutDataTypeStr=double  SampleTime=1/44100
  Multiply : Product  OutDataTypeStr=double  LockScale=on
  Multiply1 : Product  OutDataTypeStr=double  LockScale=on
  Multiply2 : Product  OutDataTypeStr=double  LockScale=on
  Rate Transition : RateTransition  OutPortSampleTime=1/44100
  Rate Transition1 : RateTransition  OutPortSampleTime=1/44100
  Out_LoD_e : Outport  OutDataTypeStr=double  SampleTime=1/44100  VectorParamsAs1DForOutWhenUnconnected=off
  wires:
  In_LoD_e/1 -> Delay/1, Multiply/2
  Delay3/1 -> Add/2
  LoD_2/1 -> Multiply1/1
  Multiply/1 -> Add/1
  Rate Transition/1 -> Delay1/1, Multiply1/2
  LoD_4/1 -> Multiply2/1
  Delay2/1 -> Add1/2
  Multiply1/1 -> Add1/1
  Multiply2/1 -> Delay2/1
  Add1/1 -> Delay3/1
  Rate Transition1/1 -> Multiply2/2
  Add/1 -> Out_LoD_e/1
  Delay1/1 -> Rate Transition1/1
  LoD_0/1 -> Multiply/1
  Delay/1 -> Rate Transition/1

== system coif1_5_Level/5th_Level_Decomp/LoD_Odd ==
  In_LoD_o : Inport  OutDataTypeStr=double  SampleTime=1/44100
  Add : Sum  AccumDataTypeStr=double  OutDataTypeStr=double  LockScale=on
  Add1 : Sum  AccumDataTypeStr=double  OutDataTypeStr=double  LockScale=on
  Delay{,1..3} (4 alike) : Delay  DelayLength=1  SampleTime=1/44100
  LoD_1 : Constant  Value=-0.07273262  OutDataTypeStr=double  SampleTime=1/44100
  LoD_3 : Constant  Value=0.85257202  OutDataTypeStr=double  SampleTime=1/44100
  LoD_5 : Constant  Value=-0.07273262  OutDataTypeStr=double  SampleTime=1/44100
  Multiply : Product  OutDataTypeStr=double  LockScale=on
  Multiply1 : Product  OutDataTypeStr=double  LockScale=on
  Multiply2 : Product  OutDataTypeStr=double  LockScale=on
  Rate Transition : RateTransition  OutPortSampleTime=1/44100
  Rate Transition1 : RateTransition  OutPortSampleTime=1/44100
  Out_LoD_o : Outport  OutDataTypeStr=double  SampleTime=1/44100  VectorParamsAs1DForOutWhenUnconnected=off
  wires:
  In_LoD_o/1 -> Delay/1, Multiply/2
  Delay3/1 -> Add/2
  LoD_3/1 -> Multiply1/1
  Delay/1 -> Rate Transition/1
  Multiply/1 -> Add/1
  Rate Transition/1 -> Delay1/1, Multiply1/2
  LoD_5/1 -> Multiply2/1
  Delay2/1 -> Add1/2
  Multiply1/1 -> Add1/1
  Multiply2/1 -> Delay2/1
  Add1/1 -> Delay3/1
  Rate Transition1/1 -> Multiply2/2
  Add/1 -> Out_LoD_o/1
  Delay1/1 -> Rate Transition1/1
  LoD_1/1 -> Multiply/1

== system coif1_5_Level/5th_Level_Recon/HiR_Even1 ==
  In_HiR_e : Inport  OutDataTypeStr=double  SampleTime=1/44100
  Add : Sum  AccumDataTypeStr=double  OutDataTypeStr=double  LockScale=on
  Add1 : Sum  AccumDataTypeStr=double  OutDataTypeStr=double  LockScale=on
  Delay{,1..3} (4 alike) : Delay  DelayLength=1  SampleTime=1/44100
  HiR_0 : Constant  Value=-0.015655728  OutDataTypeStr=double  SampleTime=1/44100
  HiR_2 : Constant  Value=0.384864847  OutDataTypeStr=double  SampleTime=1/44100
  HiR_4 : Constant  Value=0.337897662  OutDataTypeStr=double  SampleTime=1/44100
  Multiply : Product  OutDataTypeStr=double  LockScale=on
  Multiply1 : Product  OutDataTypeStr=double  LockScale=on
  Multiply2 : Product  OutDataTypeStr=double  LockScale=on
  Rate Transition : RateTransition  OutPortSampleTime=1/44100
  Rate Transition1 : RateTransition  OutPortSampleTime=1/44100
  Out_HiR_e : Outport  OutDataTypeStr=double  SampleTime=1/44100  VectorParamsAs1DForOutWhenUnconnected=off
  wires:
  In_HiR_e/1 -> Multiply/2, Delay/1
  Delay/1 -> Rate Transition/1
  Delay3/1 -> Add/2
  Multiply/1 -> Add/1
  HiR_0/1 -> Multiply/1
  HiR_2/1 -> Multiply1/1
  Rate Transition/1 -> Delay1/1, Multiply1/2
  Add/1 -> Out_HiR_e/1
  Delay1/1 -> Rate Transition1/1
  Rate Transition1/1 -> Multiply2/2
  Multiply2/1 -> Delay2/1
  Delay2/1 -> Add1/2
  Multiply1/1 -> Add1/1
  Add1/1 -> Delay3/1
  HiR_4/1 -> Multiply2/1

== system coif1_5_Level/5th_Level_Recon/HiR_Odd1 ==
  In_HiR_o : Inport  OutDataTypeStr=double  SampleTime=1/44100
  Add1 : Sum  AccumDataTypeStr=double  OutDataTypeStr=double  LockScale=on
  Add2 : Sum  AccumDataTypeStr=double  OutDataTypeStr=double  LockScale=on
  Delay{1..2,4..5} (4 alike) : Delay  DelayLength=1  SampleTime=1/44100
  HiR_1 : Constant  Value=0.07273262  OutDataTypeStr=double  SampleTime=1/44100
  HiR_3 : Constant  Value=-0.85257202  OutDataTypeStr=double  SampleTime=1/44100
  HiR_5 : Constant  Value=0.07273262  OutDataTypeStr=double  SampleTime=1/44100
  Multiply2 : Product  OutDataTypeStr=double  LockScale=on
  Multiply3 : Product  OutDataTypeStr=double  LockScale=on
  Multiply4 : Product  OutDataTypeStr=double  LockScale=on
  Rate Transition1 : RateTransition  OutPortSampleTime=1/44100
  Rate Transition2 : RateTransition  OutPortSampleTime=1/44100
  Out_HiR_o : Outport  OutDataTypeStr=double  SampleTime=1/44100  VectorParamsAs1DForOutWhenUnconnected=off
  wires:
  HiR_5/1 -> Multiply4/1
  Add1/1 -> Out_HiR_o/1
  Rate Transition2/1 -> Multiply4/2
  Rate Transition1/1 -> Delay2/1, Multiply3/2
  Multiply4/1 -> Delay4/1
  Add2/1 -> Delay5/1
  Multiply3/1 -> Add2/1
  Delay4/1 -> Add2/2
  Multiply2/1 -> Add1/1
  Delay2/1 -> Rate Transition2/1
  In_HiR_o/1 -> Multiply2/2, Delay1/1
  Delay1/1 -> Rate Transition1/1
  Delay5/1 -> Add1/2
  HiR_1/1 -> Multiply2/1
  HiR_3/1 -> Multiply3/1

== system coif1_5_Level/5th_Level_Recon/LoR_Even1 ==
  In_LoR_e : Inport  OutDataTypeStr=double  SampleTime=1/44100
  Add1 : Sum  AccumDataTypeStr=double  OutDataTypeStr=double  LockScale=on
  Add2 : Sum  AccumDataTypeStr=double  OutDataTypeStr=double  LockScale=on
  Delay{1..2,4..5} (4 alike) : Delay  DelayLength=1  SampleTime=1/44100
  LoR_0 : Constant  Value=-0.07273262  OutDataTypeStr=double  SampleTime=1/44100
  LoR_2 : Constant  Value=0.85257202  OutDataTypeStr=double  SampleTime=1/44100
  LoR_4 : Constant  Value=-0.07273262  OutDataTypeStr=double  SampleTime=1/44100
  Multiply2 : Product  OutDataTypeStr=double  LockScale=on
  Multiply3 : Product  OutDataTypeStr=double  LockScale=on
  Multiply4 : Product  OutDataTypeStr=double  LockScale=on
  Rate Transition1 : RateTransition  OutPortSampleTime=1/44100
  Rate Transition2 : RateTransition  OutPortSampleTime=1/44100
  Out_LoR_e : Outport  OutDataTypeStr=double  SampleTime=1/44100  VectorParamsAs1DForOutWhenUnconnected=off
  wires:
  Add2/1 -> Delay5/1
  Delay2/1 -> Rate Transition2/1
  Add1/1 -> Out_LoR_e/1
  Multiply3/1 -> Add2/1
  Delay5/1 -> Add1/2
  Delay1/1 -> Rate Transition1/1
  Multiply2/1 -> Add1/1
  Delay4/1 -> Add2/2
  Multiply4/1 -> Delay4/1
  Rate Transition2/1 -> Multiply4/2
  In_LoR_e/1 -> Multiply2/2, Delay1/1
  Rate Transition1/1 -> Delay2/1, Multiply3/2
  LoR_4/1 -> Multiply4/1
  LoR_2/1 -> Multiply3/1
  LoR_0/1 -> Multiply2/1

== system coif1_5_Level/5th_Level_Recon/LoR_Odd1 ==
  In_LoR_o : Inport  OutDataTypeStr=double  SampleTime=1/44100
  Add1 : Sum  AccumDataTypeStr=double  OutDataTypeStr=double  LockScale=on
  Add2 : Sum  AccumDataTypeStr=double  OutDataTypeStr=double  LockScale=on
  Delay{1..2,4..5} (4 alike) : Delay  DelayLength=1  SampleTime=1/44100
  LoR_1 : Constant  Value=0.337897662  OutDataTypeStr=double  SampleTime=1/44100
  LoR_3 : Constant  Value=0.384864847  OutDataTypeStr=double  SampleTime=1/44100
  LoR_5 : Constant  Value=-0.015655728  OutDataTypeStr=double  SampleTime=1/44100
  Multiply2 : Product  OutDataTypeStr=double  LockScale=on
  Multiply3 : Product  OutDataTypeStr=double  LockScale=on
  Multiply4 : Product  OutDataTypeStr=double  LockScale=on
  Rate Transition1 : RateTransition  OutPortSampleTime=1/44100
  Rate Transition2 : RateTransition  OutPortSampleTime=1/44100
  Out_HiR_o : Outport  OutDataTypeStr=double  SampleTime=1/44100  VectorParamsAs1DForOutWhenUnconnected=off
  wires:
  LoR_5/1 -> Multiply4/1
  In_LoR_o/1 -> Multiply2/2, Delay1/1
  LoR_3/1 -> Multiply3/1
  Delay2/1 -> Rate Transition2/1
  Add2/1 -> Delay5/1
  Multiply3/1 -> Add2/1
  Multiply2/1 -> Add1/1
  Delay4/1 -> Add2/2
  Rate Transition1/1 -> Delay2/1, Multiply3/2
  LoR_1/1 -> Multiply2/1
  Delay5/1 -> Add1/2
  Rate Transition2/1 -> Multiply4/2
  Delay1/1 -> Rate Transition1/1
  Multiply4/1 -> Delay4/1
  Add1/1 -> Out_HiR_o/1

== system coif1_5_Level/Threshold_Estimator/Absolute_Value1 ==
  Signal_w4 : Inport  OutDataTypeStr=double  SampleTime=1/44100
  Absolute_Switch : Switch  Threshold=1  OutDataTypeStr=double
  Constant295 : Constant  Value=0  OutDataTypeStr=double  SampleTime=1/44100
  Gain2 : Gain  Gain=-1  ParamDataTypeStr=double  OutDataTypeStr=double
  Relational Operator2 : RelationalOperator  Operator=<  OutDataTypeStr=boolean  RndMeth=Simplest
  Out_Abs : Outport  OutDataTypeStr=double  SampleTime=1/44100  VectorParamsAs1DForOutWhenUnconnected=off
  wires:
  Absolute_Switch/1 -> Out_Abs/1
  Relational Operator2/1 -> Absolute_Switch/2
  Gain2/1 -> Absolute_Switch/1
  Signal_w4/1 -> Absolute_Switch/3, Relational Operator2/1, Gain2/1
  Constant295/1 -> Relational Operator2/2

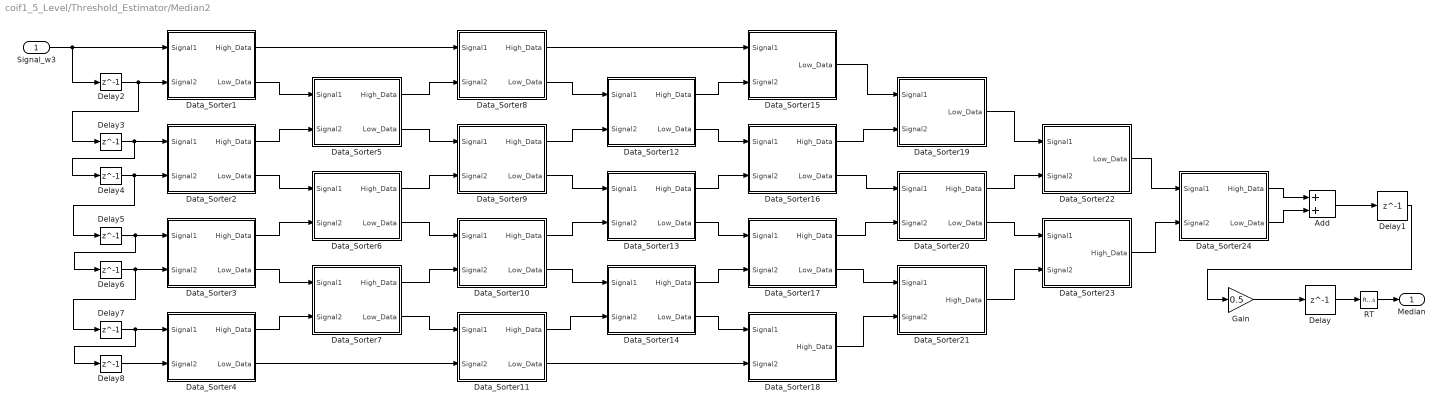
== system coif1_5_Level/Threshold_Estimator/Median2 ==
  Signal_w3 : Inport  OutDataTypeStr=double  SampleTime=1/44100
  Add : Sum  AccumDataTypeStr=double  OutDataTypeStr=double
  Data_Sorter1 : Subsystem
  Data_Sorter10 : Subsystem
  Data_Sorter11 : Subsystem
  Data_Sorter12 : Subsystem
  Data_Sorter13 : Subsystem
  Data_Sorter14 : Subsystem
  Data_Sorter15 : Subsystem
  Data_Sorter16 : Subsystem
  Data_Sorter17 : Subsystem
  Data_Sorter18 : Subsystem
  Data_Sorter19 : Subsystem
  Data_Sorter2 : Subsystem
  Data_Sorter20 : Subsystem
  Data_Sorter21 : Subsystem
  Data_Sorter22 : Subsystem
  Data_Sorter23 : Subsystem
  Data_Sorter24 : Subsystem
  Data_Sorter3 : Subsystem
  Data_Sorter4 : Subsystem
  Data_Sorter5 : Subsystem
  Data_Sorter6 : Subsystem
  Data_Sorter7 : Subsystem
  Data_Sorter8 : Subsystem
  Data_Sorter9 : Subsystem
  Delay{,1..8} (9 alike) : Delay  DelayLength=1  SampleTime=1/44100
  Gain : Gain  Gain=0.5  ParamDataTypeStr=double  OutDataTypeStr=double
  RT : RateTransition  OutPortSampleTime=1/44100
  Median : Outport  OutDataTypeStr=double  SampleTime=1/44100  VectorParamsAs1DForOutWhenUnconnected=off
  wires:
  Data_Sorter4/1(High_Data) -> Data_Sorter7/2(Signal2)
  Delay3/1 -> Data_Sorter2/1(Signal1), Delay4/1
  Signal_w3/1 -> Data_Sorter1/1(Signal1), Delay2/1
  Data_Sorter10/1(High_Data) -> Data_Sorter13/2(Signal2)
  Data_Sorter23/1(High_Data) -> Data_Sorter24/2(Signal2)
  Data_Sorter12/2(Low_Data) -> Data_Sorter16/1(Signal1)
  Delay2/1 -> Delay3/1, Data_Sorter1/2(Signal2)
  Data_Sorter5/1(High_Data) -> Data_Sorter8/2(Signal2)
  Delay/1 -> RT/1
  Data_Sorter15/1(Low_Data) -> Data_Sorter19/1(Signal1)
  Add/1 -> Delay1/1
  Data_Sorter7/2(Low_Data) -> Data_Sorter11/1(Signal1)
  Data_Sorter24/1(High_Data) -> Add/1
  Data_Sorter1/2(Low_Data) -> Data_Sorter5/1(Signal1)
  Data_Sorter3/1(High_Data) -> Data_Sorter6/2(Signal2)
  Data_Sorter22/1(Low_Data) -> Data_Sorter24/1(Signal1)
  Data_Sorter2/1(High_Data) -> Data_Sorter5/2(Signal2)
  Data_Sorter10/2(Low_Data) -> Data_Sorter14/1(Signal1)
  Delay1/1 -> Gain/1
  Data_Sorter17/2(Low_Data) -> Data_Sorter21/1(Signal1)
  Data_Sorter21/1(High_Data) -> Data_Sorter23/2(Signal2)
  Data_Sorter7/1(High_Data) -> Data_Sorter10/2(Signal2)
  Delay4/1 -> Data_Sorter2/2(Signal2), Delay5/1
  Data_Sorter16/1(High_Data) -> Data_Sorter19/2(Signal2)
  Data_Sorter20/1(High_Data) -> Data_Sorter22/2(Signal2)
  Data_Sorter16/2(Low_Data) -> Data_Sorter20/1(Signal1)
  Data_Sorter3/2(Low_Data) -> Data_Sorter7/1(Signal1)
  Data_Sorter2/2(Low_Data) -> Data_Sorter6/1(Signal1)
  Data_Sorter6/2(Low_Data) -> Data_Sorter10/1(Signal1)
  Data_Sorter19/1(Low_Data) -> Data_Sorter22/1(Signal1)
  Data_Sorter12/1(High_Data) -> Data_Sorter15/2(Signal2)
  Data_Sorter5/2(Low_Data) -> Data_Sorter9/1(Signal1)
  Data_Sorter24/2(Low_Data) -> Add/2
  Data_Sorter17/1(High_Data) -> Data_Sorter20/2(Signal2)
  Data_Sorter13/1(High_Data) -> Data_Sorter16/2(Signal2)
  Data_Sorter11/1(High_Data) -> Data_Sorter14/2(Signal2)
  Delay8/1 -> Data_Sorter4/2(Signal2)
  Data_Sorter8/2(Low_Data) -> Data_Sorter12/1(Signal1)
  Delay6/1 -> Data_Sorter3/2(Signal2), Delay7/1
  Data_Sorter9/2(Low_Data) -> Data_Sorter13/1(Signal1)
  Data_Sorter4/2(Low_Data) -> Data_Sorter11/2(Signal2)
  Data_Sorter9/1(High_Data) -> Data_Sorter12/2(Signal2)
  Data_Sorter14/2(Low_Data) -> Data_Sorter18/1(Signal1)
  Delay5/1 -> Data_Sorter3/1(Signal1), Delay6/1
  Delay7/1 -> Data_Sorter4/1(Signal1), Delay8/1
  Data_Sorter1/1(High_Data) -> Data_Sorter8/1(Signal1)
  Data_Sorter8/1(High_Data) -> Data_Sorter15/1(Signal1)
  Data_Sorter14/1(High_Data) -> Data_Sorter17/2(Signal2)
  Data_Sorter6/1(High_Data) -> Data_Sorter9/2(Signal2)
  Data_Sorter20/2(Low_Data) -> Data_Sorter23/1(Signal1)
  Data_Sorter11/2(Low_Data) -> Data_Sorter18/2(Signal2)
  Data_Sorter13/2(Low_Data) -> Data_Sorter17/1(Signal1)
  Gain/1 -> Delay/1
  Data_Sorter18/1(High_Data) -> Data_Sorter21/2(Signal2)
  RT/1 -> Median/1

== system coif1_5_Level/Threshold_Estimator/Median2/Data_Sorter1 ==
  Signal1 : Inport  OutDataTypeStr=double  SampleTime=1/44100
  Signal2 : Inport  Port=2  OutDataTypeStr=double  SampleTime=1/44100
  Data_Sorter_Switch : Switch  OutDataTypeStr=double
  Data_Sorter_Switch1 : Switch  Threshold=1  OutDataTypeStr=double
  Delay1 : Delay  DelayLength=1  SampleTime=1/44100
  Delay2 : Delay  DelayLength=1  SampleTime=1/44100
  Relational Operator2 : RelationalOperator  Operator=<  OutDataTypeStr=boolean  RndMeth=Simplest
  High_Data : Outport  OutDataTypeStr=double  SampleTime=1/44100  VectorParamsAs1DForOutWhenUnconnected=off
  Low_Data : Outport  Port=2  OutDataTypeStr=double  SampleTime=1/44100  VectorParamsAs1DForOutWhenUnconnected=off
  wires:
  Signal1/1 -> Data_Sorter_Switch/3, Data_Sorter_Switch/1, Relational Operator2/1
  Relational Operator2/1 -> Data_Sorter_Switch1/2, Data_Sorter_Switch/2
  Signal2/1 -> Data_Sorter_Switch1/1, Data_Sorter_Switch1/3, Relational Operator2/2
  Data_Sorter_Switch1/1 -> Delay2/1
  Delay2/1 -> Low_Data/1
  Data_Sorter_Switch/1 -> Delay1/1
  Delay1/1 -> High_Data/1

== system coif1_5_Level/Threshold_Estimator/Median2/Data_Sorter10 ==
  Signal1 : Inport  OutDataTypeStr=double  SampleTime=1/44100
  Signal2 : Inport  Port=2  OutDataTypeStr=double  SampleTime=1/44100
  Data_Sorter_Switch : Switch  OutDataTypeStr=double
  Data_Sorter_Switch1 : Switch  Threshold=1  OutDataTypeStr=double
  Delay1 : Delay  DelayLength=1  SampleTime=1/44100
  Delay2 : Delay  DelayLength=1  SampleTime=1/44100
  Relational Operator2 : RelationalOperator  Operator=<  OutDataTypeStr=boolean  RndMeth=Simplest
  High_Data : Outport  OutDataTypeStr=double  SampleTime=1/44100  VectorParamsAs1DForOutWhenUnconnected=off
  Low_Data : Outport  Port=2  OutDataTypeStr=double  SampleTime=1/44100  VectorParamsAs1DForOutWhenUnconnected=off
  wires:
  Signal1/1 -> Data_Sorter_Switch/3, Data_Sorter_Switch/1, Relational Operator2/1
  Relational Operator2/1 -> Data_Sorter_Switch1/2, Data_Sorter_Switch/2
  Signal2/1 -> Data_Sorter_Switch1/1, Data_Sorter_Switch1/3, Relational Operator2/2
  Data_Sorter_Switch1/1 -> Delay2/1
  Delay2/1 -> Low_Data/1
  Data_Sorter_Switch/1 -> Delay1/1
  Delay1/1 -> High_Data/1

== system coif1_5_Level/Threshold_Estimator/Median2/Data_Sorter11 ==
  Signal1 : Inport  OutDataTypeStr=double  SampleTime=1/44100
  Signal2 : Inport  Port=2  OutDataTypeStr=double  SampleTime=1/44100
  Data_Sorter_Switch : Switch  OutDataTypeStr=double
  Data_Sorter_Switch1 : Switch  Threshold=1  OutDataTypeStr=double
  Delay1 : Delay  DelayLength=1  SampleTime=1/44100
  Delay2 : Delay  DelayLength=1  SampleTime=1/44100
  Relational Operator2 : RelationalOperator  Operator=<  OutDataTypeStr=boolean  RndMeth=Simplest
  High_Data : Outport  OutDataTypeStr=double  SampleTime=1/44100  VectorParamsAs1DForOutWhenUnconnected=off
  Low_Data : Outport  Port=2  OutDataTypeStr=double  SampleTime=1/44100  VectorParamsAs1DForOutWhenUnconnected=off
  wires:
  Signal1/1 -> Data_Sorter_Switch/3, Data_Sorter_Switch/1, Relational Operator2/1
  Relational Operator2/1 -> Data_Sorter_Switch1/2, Data_Sorter_Switch/2
  Signal2/1 -> Data_Sorter_Switch1/1, Data_Sorter_Switch1/3, Relational Operator2/2
  Data_Sorter_Switch1/1 -> Delay2/1
  Delay2/1 -> Low_Data/1
  Data_Sorter_Switch/1 -> Delay1/1
  Delay1/1 -> High_Data/1

== system coif1_5_Level/Threshold_Estimator/Median2/Data_Sorter12 ==
  Signal1 : Inport  OutDataTypeStr=double  SampleTime=1/44100
  Signal2 : Inport  Port=2  OutDataTypeStr=double  SampleTime=1/44100
  Data_Sorter_Switch : Switch  OutDataTypeStr=double
  Data_Sorter_Switch1 : Switch  Threshold=1  OutDataTypeStr=double
  Delay1 : Delay  DelayLength=1  SampleTime=1/44100
  Delay2 : Delay  DelayLength=1  SampleTime=1/44100
  Relational Operator2 : RelationalOperator  Operator=<  OutDataTypeStr=boolean  RndMeth=Simplest
  High_Data : Outport  OutDataTypeStr=double  SampleTime=1/44100  VectorParamsAs1DForOutWhenUnconnected=off
  Low_Data : Outport  Port=2  OutDataTypeStr=double  SampleTime=1/44100  VectorParamsAs1DForOutWhenUnconnected=off
  wires:
  Signal1/1 -> Data_Sorter_Switch/3, Data_Sorter_Switch/1, Relational Operator2/1
  Relational Operator2/1 -> Data_Sorter_Switch1/2, Data_Sorter_Switch/2
  Signal2/1 -> Data_Sorter_Switch1/1, Data_Sorter_Switch1/3, Relational Operator2/2
  Data_Sorter_Switch1/1 -> Delay2/1
  Delay2/1 -> Low_Data/1
  Data_Sorter_Switch/1 -> Delay1/1
  Delay1/1 -> High_Data/1
